simulink model "MAXMathsWithDTInt"  (R2017a)
settings: Solver=FixedStepAuto  StartTime=0.0  StopTime=5  FixedStep=tstep  MaxStep=tstep  RelTol=1e-3
InitFcn:
  | initMAX;
StopFcn:
  | plotMAX;
undefined symbols (not defined in the file or in its folder): DiscIntNeverNeededParam, m, problem, tstep
settings Model: Creator=yn15  LastModifiedBy=daw15
settings SolverCC: SolverResetMethod=Robust
settings OptimizationCC: LifeSpan=inf
settings DebuggingCC: SFUnexpectedBacktrackingDiag=warning  SFNoUnconditionalDefaultTransitionDiag=warning  SFExecutionAtInitializationDiag=none
settings GRTTargetCC: TargetLangStandard=C89/C90 (ANSI)
settings ConfigComp: CovMetricSettings=dw  CovHtmlReporting=on  CovSaveCumulativeToWorkspaceVar=on  CovSaveSingleToWorkspaceVar=on  CovExternalEMLEnable=off

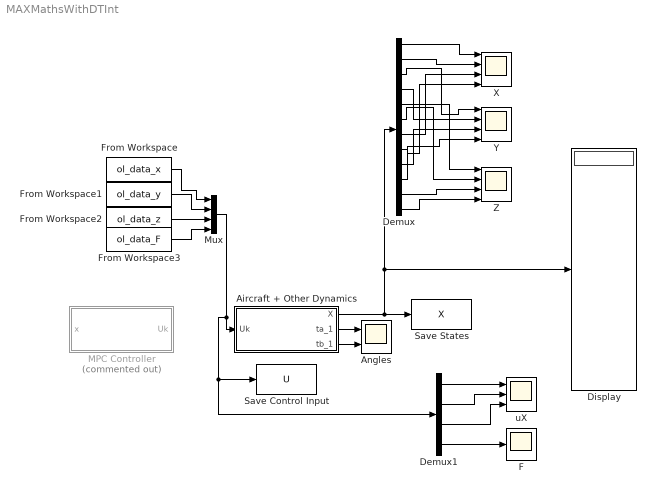
== system MAXMathsWithDTInt ==
  Aircraft + Other Dynamics : Subsystem
  Angles : Scope  NumInputPorts=2
  Demux : Demux  Outputs=12
  Demux1 : Demux
  Display : Display
  F : Scope
  From Workspace : FromWorkspace  VariableName=ol_data_x  SampleTime=0
  From Workspace1 : FromWorkspace  VariableName=ol_data_y  SampleTime=0
  From Workspace2 : FromWorkspace  VariableName=ol_data_z  SampleTime=0
  From Workspace3 : FromWorkspace  VariableName=ol_data_F  SampleTime=0
  "MPC Controller " : Subsystem  Commented=on
  Mux : Mux
  Save Control Input : ToWorkspace  VariableName=U  SampleTime=-1
      settings: Save2DSignal=2-D array (concatenate along first dimension)
  Save States : ToWorkspace  VariableName=X  SaveFormat=Timeseries  SampleTime=-1
  X : Scope  NumInputPorts=4
  Y : Scope  NumInputPorts=4
  Z : Scope  NumInputPorts=4
  uX : Scope  NumInputPorts=3
  wires:
  Aircraft + Other Dynamics/1(X) -> Demux/1, Display/1, Save States/1
  Demux1/3 -> uX/3
  Demux1/4 -> F/1
  Demux/1 -> X/1
  Demux/2 -> X/2
  Demux/3 -> Y/1
  Demux/4 -> Y/2
  Demux/5 -> Z/1
  Demux/6 -> Z/2
  Demux/7 -> X/3
  Demux/8 -> X/4
  Demux/9 -> Y/3
  Demux/10 -> Y/4
  Demux/11 -> Z/3
  Demux/12 -> Z/4
  Aircraft + Other Dynamics/2(ta_1) -> Angles/1
  Aircraft + Other Dynamics/3(tb_1) -> Angles/2
  Demux1/1 -> uX/1
  Demux1/2 -> uX/2
  From Workspace/1 -> Mux/1
  Mux/1 -> Demux1/1, Save Control Input/1, Aircraft + Other Dynamics/1(Uk)
  From Workspace1/1 -> Mux/2
  From Workspace2/1 -> Mux/3
  From Workspace3/1 -> Mux/4

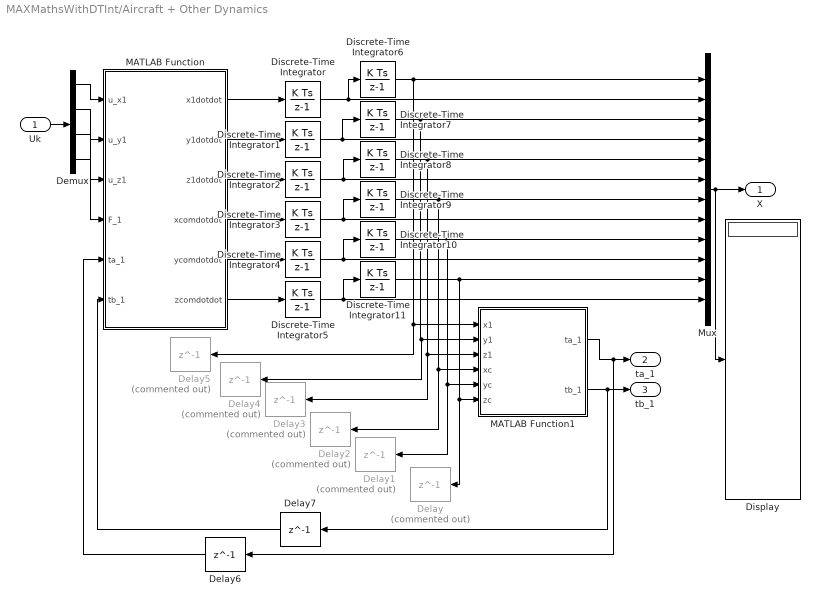
== system MAXMathsWithDTInt/Aircraft + Other Dynamics ==
  Uk : Inport
  Delay : Delay  Commented=on  DelayLength=1  InitialCondition=1
  Delay1 : Delay  Commented=on  DelayLength=1
  Delay2 : Delay  Commented=on  DelayLength=1  InitialCondition=2.1
  Delay3 : Delay  Commented=on  DelayLength=1  InitialCondition=2.2
  Delay4 : Delay  Commented=on  DelayLength=1
  Delay5 : Delay  Commented=on  DelayLength=1  InitialCondition=2.1
  Delay6 : Delay  DelayLength=1  InitialCondition=0  SampleTime=tstep
  Delay7 : Delay  DelayLength=1  InitialCondition=0  SampleTime=tstep
  Demux : Demux
  Discrete-Time Integrator{,1..5,7,10} (8 alike) : DiscreteIntegrator  gainval=1  SampleTime=tstep  ICPrevOutput=DiscIntNeverNeededParam  ICPrevScaledInput=DiscIntNeverNeededParam
  Discrete-Time Integrator11 : DiscreteIntegrator  gainval=1  InitialCondition=1  SampleTime=tstep  ICPrevOutput=DiscIntNeverNeededParam  ICPrevScaledInput=DiscIntNeverNeededParam
  Discrete-Time Integrator6 : DiscreteIntegrator  gainval=1  InitialCondition=2.1  SampleTime=tstep  ICPrevOutput=DiscIntNeverNeededParam  ICPrevScaledInput=DiscIntNeverNeededParam
  Discrete-Time Integrator8 : DiscreteIntegrator  gainval=1  InitialCondition=2.2  SampleTime=tstep  ICPrevOutput=DiscIntNeverNeededParam  ICPrevScaledInput=DiscIntNeverNeededParam
  Discrete-Time Integrator9 : DiscreteIntegrator  gainval=1  InitialCondition=2.1  SampleTime=tstep  ICPrevOutput=DiscIntNeverNeededParam  ICPrevScaledInput=DiscIntNeverNeededParam
  Display : Display
  MATLAB Function : MATLAB Function  TreatAsAtomicUnit=on
  MATLAB Function1 : MATLAB Function  TreatAsAtomicUnit=on
  Mux : Mux  Inputs=12
  X : Outport
  ta_1 : Outport  Port=2
  tb_1 : Outport  Port=3
  wires:
  Discrete-Time Integrator/1 -> Discrete-Time Integrator6/1, Mux/2
  Discrete-Time Integrator1/1 -> Discrete-Time Integrator7/1, Mux/4
  Discrete-Time Integrator2/1 -> Discrete-Time Integrator8/1, Mux/6
  Discrete-Time Integrator3/1 -> Discrete-Time Integrator9/1, Mux/8
  Discrete-Time Integrator6/1 -> Delay5/1, MATLAB Function1/1(x1), Mux/1
  Discrete-Time Integrator7/1 -> Delay4/1, MATLAB Function1/2(y1), Mux/3
  Discrete-Time Integrator8/1 -> Delay3/1, MATLAB Function1/3(z1), Mux/5
  Discrete-Time Integrator9/1 -> Delay2/1, MATLAB Function1/4(xc), Mux/7
  Uk/1 -> Demux/1
  Demux/1 -> MATLAB Function/1(u_x1)
  Demux/2 -> MATLAB Function/2(u_y1)
  Demux/3 -> MATLAB Function/3(u_z1)
  Demux/4 -> MATLAB Function/4(F_1)
  Discrete-Time Integrator4/1 -> Discrete-Time Integrator10/1, Mux/10
  Discrete-Time Integrator5/1 -> Discrete-Time Integrator11/1, Mux/12
  Discrete-Time Integrator10/1 -> Delay1/1, MATLAB Function1/5(yc), Mux/9
  Discrete-Time Integrator11/1 -> Delay/1, MATLAB Function1/6(zc), Mux/11
  MATLAB Function/1(x1dotdot) -> Discrete-Time Integrator/1
  MATLAB Function/2(y1dotdot) -> Discrete-Time Integrator1/1
  MATLAB Function/3(z1dotdot) -> Discrete-Time Integrator2/1
  MATLAB Function/4(xcomdotdot) -> Discrete-Time Integrator3/1
  MATLAB Function/5(ycomdotdot) -> Discrete-Time Integrator4/1
  MATLAB Function/6(zcomdotdot) -> Discrete-Time Integrator5/1
  MATLAB Function1/1(ta_1) -> Delay6/1, ta_1/1
  MATLAB Function1/2(tb_1) -> Delay7/1, tb_1/1
  Mux/1 -> X/1, Display/1
  Delay6/1 -> MATLAB Function/5(ta_1)
  Delay7/1 -> MATLAB Function/6(tb_1)

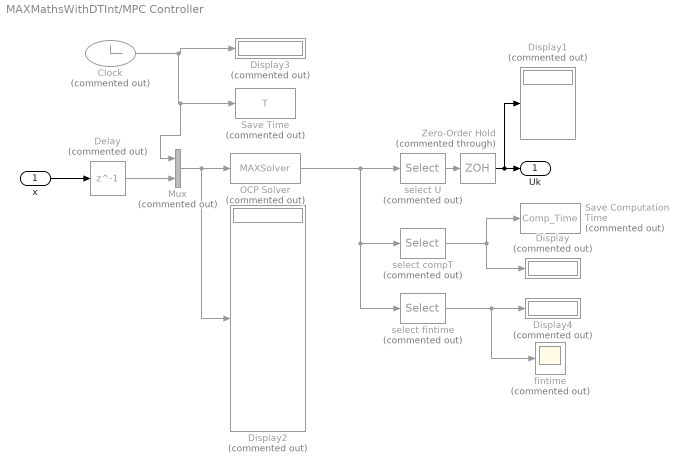
== system MAXMathsWithDTInt/MPC Controller  ==
  x : Inport
  Clock : Clock  Commented=on
  Delay : Delay  Commented=on  DelayLength=1  InitialCondition=[problem.states.x0]
  Display{,1..4} (5 alike) : Display  Commented=on
  Mux : Mux  Commented=on  Inputs=2
  OCP Solver : MATLABFcn  Commented=on  MATLABFcn=MAXSolver  OutputDimensions=m+2
  "Save Computation Time " : ToWorkspace  Commented=on  VariableName=Comp_Time  SampleTime=tstep
      settings: Save2DSignal=2-D array (concatenate along first dimension)
  Save Time : ToWorkspace  Commented=on  VariableName=T  SampleTime=-1
      settings: Save2DSignal=2-D array (concatenate along first dimension)
  Zero-Order Hold : ZeroOrderHold  Commented=through  SampleTime=tstep
  fintime : Scope  Commented=on
  select U : Selector  Commented=on  IndexOptions=Index vector (dialog)  Indices=3:m+2  OutputSizes=1
  select compT : Selector  Commented=on  IndexOptions=Index vector (dialog)  Indices=2  OutputSizes=1
  select fintime : Selector  Commented=on  IndexOptions=Index vector (dialog)  Indices=1  OutputSizes=1
  Uk : Outport
  wires:
  OCP Solver/1 -> select U/1, select fintime/1, select compT/1
  select compT/1 -> "Save Computation Time "/1, Display/1
  Mux/1 -> Display2/1, OCP Solver/1
  select fintime/1 -> fintime/1, Display4/1
  Delay/1 -> Mux/2
  Clock/1 -> Mux/1, Save Time/1, Display3/1
  select U/1 -> Zero-Order Hold/1
  Zero-Order Hold/1 -> Display1/1, Uk/1
  x/1 -> Delay/1

== matlab function MAXMathsWithDTInt/Aircraft + Other Dynamics/MATLAB Function1 ==
  data: x1 input; ta_1 output; y1 input; z1 input; xc input; yc input; zc input; tb_1 output
function [ta_1,tb_1] = updateAngles(x1,y1,z1,xc,yc,zc)

ta_1 = (x1-xc)/(z1-zc);
tb_1 = (y1-yc)/(z1-zc);

== matlab function MAXMathsWithDTInt/Aircraft + Other Dynamics/MATLAB Function ==
  data: x1dotdot output; y1dotdot output; z1dotdot output; u_x1 input; u_y1 input; u_z1 input; F_1 input; xcomdotdot output; ycomdotdot output; zcomdotdot output; ta_1 input; tb_1 input
function [x1dotdot,y1dotdot,z1dotdot,xcomdotdot,ycomdotdot,zcomdotdot]= dynamics(u_x1,u_y1,u_z1,F_1,ta_1,tb_1)

m_ag = 0.81;
m_pl = 2;
g = 9.81;

% ta_1 = (x1-xc)/(z1-zc);
% tb_1 = (y1-yc)/(z1-zc);

x1dotdot =  (1/m_ag)*(u_x1 -F_1.*ta_1); %x1..
y1dotdot =  (1/m_ag)*(u_y1 -F_1.*tb_1); %y1..
z1dotdot =  (1/m_ag)*(u_z1 -F_1 -m_ag*g); %z1..
xcomdotdot =  (1/m_pl)*(F_1.*ta_1);%xcom..
ycomdotdot = (1/m_pl)*(F_1.*tb_1);%ycom..
zcomdotdot = (1/m_pl)*(F_1 - m_pl.*g);%zcom..
